simulink model "vaja_4"  (R2024b)
settings: Solver=VariableStepAuto  StartTime=0.0  StopTime=sim_time  MaxStep=0.01  RelTol=1e-3
values from neighbouring files (symbols this model uses):
  k0 = 8/3    (= 2.66666666667)    [vaja_4.m]
  k1 = tocke_stabilnosti(:, 1)    [vaja_4.m]
  k2 = tocke_stabilnosti(:, 2)    [vaja_4.m]
settings Model: Creator=gaspers  LastModifiedBy=gaspers

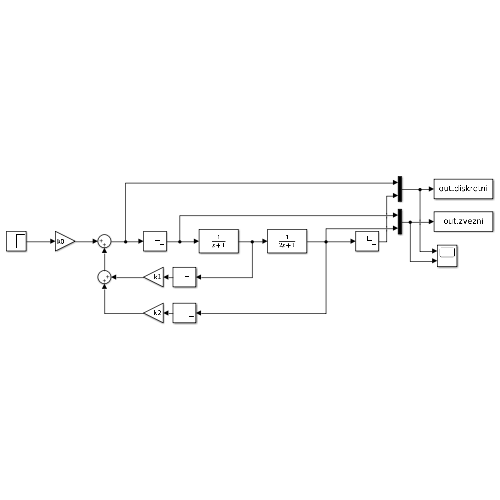
[thumbnail: Simulink's stored preview of the top-level diagram]
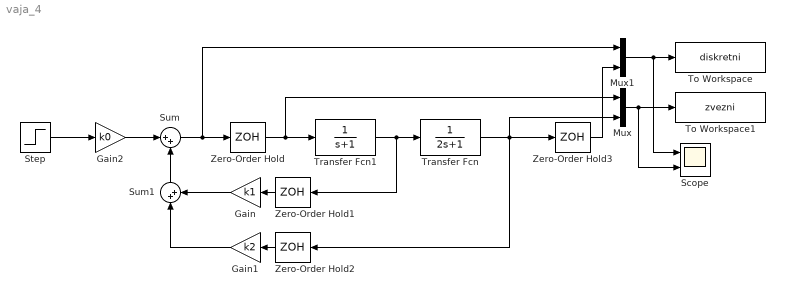
== system vaja_4 ==
  Gain : Gain  Gain=k1
  Gain1 : Gain  Gain=k2
  Gain2 : Gain  Gain=k0
  Mux : Mux  Inputs=2
  Mux1 : Mux  Inputs=2
  Scope : Scope  NumInputPorts=2
  Step : Step  SampleTime=1.3863
  Sum : Sum  Inputs=|++
  Sum1 : Sum  Inputs=|++
  To Workspace : ToWorkspace  VariableName=diskretni  SaveFormat=Timeseries  SampleTime=-1
  To Workspace1 : ToWorkspace  VariableName=zvezni  SaveFormat=Timeseries  SampleTime=-1
  Transfer Fcn : TransferFcn  Denominator=[2 1]
  Transfer Fcn1 : TransferFcn  Denominator=[1 1]
  Zero-Order Hold{,1..3} (4 alike) : ZeroOrderHold  SampleTime=1.3863
  wires:
  Zero-Order Hold/1 -> Mux/1, Transfer Fcn1/1
  Sum/1 -> Mux1/1, Zero-Order Hold/1
  Gain/1 -> Sum1/2
  Sum1/1 -> Sum/2
  Gain1/1 -> Sum1/1
  Gain2/1 -> Sum/1
  Step/1 -> Gain2/1
  Zero-Order Hold1/1 -> Gain/1
  Transfer Fcn1/1 -> Zero-Order Hold1/1, Transfer Fcn/1
  Zero-Order Hold2/1 -> Gain1/1
  Transfer Fcn/1 -> Zero-Order Hold2/1, Mux/2, Zero-Order Hold3/1
  Zero-Order Hold3/1 -> Mux1/2
  Mux/1 -> To Workspace1/1, Scope/2
  Mux1/1 -> Scope/1, To Workspace/1
